simulink model "week1Prob1model"  (R2020a)
settings: Solver=VariableStepAuto  StartTime=0.0  StopTime=10.0  RelTol=1e-3
model workspace (MAT data in the model file):
  B1 = Simulink.Parameter
  B1.Value = 50
  B1.DataType = 'auto'
  B1.Dimensions = [1 1]
  K1 = Simulink.Parameter
  K1.Value = 50
  K1.DataType = 'auto'
  K1.Dimensions = [1 1]
  K12 = Simulink.Parameter
  K12.Value = 29.6481564748
  K12.DataType = 'auto'
  K12.Dimensions = [1 1]
  M1 = Simulink.Parameter
  M1.Value = 100
  M1.DataType = 'auto'
  M1.Dimensions = [1 1]
  M2 = Simulink.Parameter
  M2.Value = 134.597222222
  M2.DataType = 'auto'
  M2.Dimensions = [1 1]
  h2r = Simulink.Parameter
  h2r.Value = 6.28318530718
  h2r.DataType = 'auto'
  h2r.Dimensions = [1 1]
  t = Simulink.Parameter
  t.Value = [0; 0.01; 0.02; 0.03; 0.04; 0.05; 0.06; 0.07; 0.08; 0.09; 0.1; 0.11; 0.12; 0.13; 0.14; 0.15; 0.16; 0.17; 0.18; 0.19; 0.2; 0.21; 0.22; 0.23; 0.24; 0.25; 0.26; 0.27; 0.28; 0.29; 0.3; 0.31; 0.32; 0.33; 0.34; 0.35; 0.36; 0.37; 0.38; 0.39; 0.4; 0.41; 0.42; 0.43; 0.44; 0.45; 0.46; 0.47; 0.48; 0.49; 0.5; 0.51; 0.52; 0.53; 0.54; 0.55; 0.56; 0.57; 0.58; 0.59; 0.6; 0.61; 0.62; 0.63; 0.64; 0.65; 0.66; 0.67; 0.68; 0.69; 0.7; 0.71; 0.72; 0.73; 0.74; 0.75; 0.76; 0.77; 0.78; 0.79; 0.8; 0.81; 0.82; 0.83; 0.84; 0.85; 0.86; 0.87; 0.88; 0.89; 0.9; 0.91; 0.92; 0.93; 0.94; 0.95; 0.96; 0.97; 0.98; 0.99; 1]
  t.DataType = 'auto'
  t.Dimensions = [101 1]
settings Model: Creator=avn19  LastModifiedBy=avn19

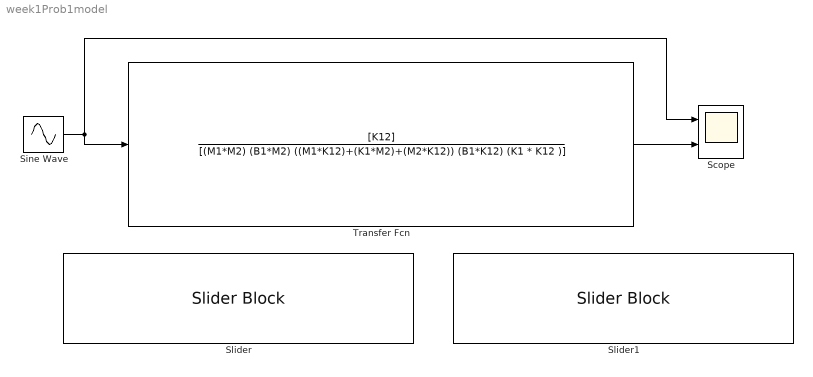
== system week1Prob1model ==
  Scope : Scope  NumInputPorts=2
  Sine Wave : Sin  Amplitude=2  Frequency=10*h2r  SampleTime=0
  Slider : SliderBlock  ScaleMax=200  TickInterval=10
  Slider1 : SliderBlock  ScaleMax=200  TickInterval=10
  Transfer Fcn : TransferFcn  Numerator=[K12]  Denominator=[(M1*M2) (B1*M2) ((M1*K12)+(K1*M2)+(M2*K12)) (B1*K12) (K1 * K12 )]
  wires:
  Sine Wave/1 -> Transfer Fcn/1, Scope/1
  Transfer Fcn/1 -> Scope/2
